simulink model "Pole_Placement_Discrete"  (R2020a)
settings: Solver=VariableStepAuto  StartTime=0.0  StopTime=10.0  RelTol=1e-3
values from neighbouring files (symbols this model uses):
  A_c = [0 1;0 0]    [Discrete_pole_placement.m]
  B_c = [0;K]    [Discrete_pole_placement.m]
  C_c = [1 0]    [Discrete_pole_placement.m]
  Con = 1    [Discrete_pole_placement.m]    (also in Pole_Placement_Integrator.m = 0; Pole_Placement_PID.m = 0)
  D_c = 0    [Discrete_pole_placement.m]
  down = -up    (= -0.10471975512)    [Discrete_pole_placement.m]    (also in Pole_Placement_PID.m = -0.0872664625997)
  K1 = place(A_d,B_d,p_d)    [Discrete_pole_placement.m]    (also in Pole_Placement_Integrator.m = place([A zeros(2,1);-C 0],[B;0],p); Pole_Placement_PID.m = 6.1486)
  L = (A_d^2+sum*A_d+prod*eye(2))*(OBS_d)^(-1)*[0;1]    [Discrete_pole_placement.m]    (also in Pole_Placement_Integrator.m = (A^2+100*A+2500*eye(2))*OBS^(-1)*[0;1])
  steady = D_d+C_d*(eye(2)-(A_d-B_d*K1))^(-1)*B_d    [Discrete_pole_placement.m]
  Ts = 0.02    [Discrete_pole_placement.m]    (also in Pole_Placement_PID.m)
  up = 6*pi/180    (= 0.10471975512)    [Discrete_pole_placement.m]    (also in Pole_Placement_PID.m = 0.0872664625997)
  x0 = 0.1    [Discrete_pole_placement.m]    (also in Pole_Placement_Integrator.m = 0.3; Pole_Placement_PID.m = 0.3)
  y0 = 0.15    [Discrete_pole_placement.m]    (also in Pole_Placement_Integrator.m = 0.3; Pole_Placement_PID.m = 0.3)
undefined symbols (not defined in the file or in its folder): A_d, B_d, C_d
settings Model: Creator=Ashraf  LastModifiedBy=hhiastt
settings DataIOCC: ReturnWorkspaceOutputs=off
settings DebuggingCC: ArithmeticOperatorsInVariantConditions=warning
settings SFSimCC: SimUseLocalCustomCode=off  CustomCodeUndefinedFunction=UseInterfaceOnly
settings RTWCC: RTWUseLocalCustomCode=off
settings CodeAppCC: StateflowObjectComments=on

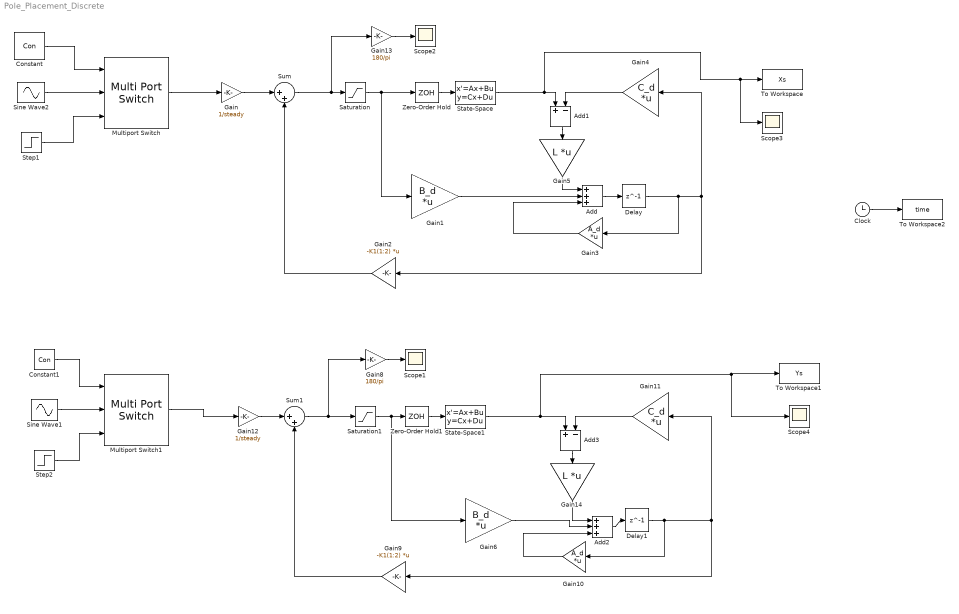
== system Pole_Placement_Discrete ==
  Add : Sum  Inputs=+++
  Add1 : Sum  Inputs=+-
  Add2 : Sum  Inputs=+++
  Add3 : Sum  Inputs=+-
  Clock : Clock
  Constant : Constant  Value=Con
  Constant1 : Constant  Value=Con
  Delay : Delay  DelayLength=1  SampleTime=Ts
  Delay1 : Delay  DelayLength=1  SampleTime=Ts
  Gain : Gain  Gain=1/steady
  Gain1 : Gain  Gain=B_d  Multiplication=Matrix(K*u)
  Gain10 : Gain  Gain=A_d  Multiplication=Matrix(K*u)
  Gain11 : Gain  Gain=C_d  Multiplication=Matrix(K*u)
  Gain12 : Gain  Gain=1/steady
  Gain13 : Gain  Gain=180/pi
  Gain14 : Gain  Gain=L  Multiplication=Matrix(K*u)
  Gain2 : Gain  Gain=-K1(1:2)  Multiplication=Matrix(K*u)
  Gain3 : Gain  Gain=A_d  Multiplication=Matrix(K*u)
  Gain4 : Gain  Gain=C_d  Multiplication=Matrix(K*u)
  Gain5 : Gain  Gain=L  Multiplication=Matrix(K*u)
  Gain6 : Gain  Gain=B_d  Multiplication=Matrix(K*u)
  Gain8 : Gain  Gain=180/pi
  Gain9 : Gain  Gain=-K1(1:2)  Multiplication=Matrix(K*u)
  Multiport Switch : MultiPortSwitch  DataPortOrder=Zero-based contiguous  Inputs=2  zeroidx=on
  Multiport Switch1 : MultiPortSwitch  DataPortOrder=Zero-based contiguous  Inputs=2  zeroidx=on
  Saturation : Saturate  UpperLimit=up  LowerLimit=down
  Saturation1 : Saturate  UpperLimit=up  LowerLimit=down
  Scope{1..4} (4 alike) : Scope
  Sine Wave1 : Sin  Amplitude=0.3  SampleTime=0
  Sine Wave2 : Sin  Amplitude=0.3  Phase=pi/2  SampleTime=Ts
  State-Space : StateSpace  A=A_c  B=B_c  C=C_c  D=D_c  InitialCondition=0
  State-Space1 : StateSpace  A=A_c  B=B_c  C=C_c  D=D_c  InitialCondition=0
  Step1 : Step  Time=0  After=x0  SampleTime=Ts
  Step2 : Step  Time=0  After=y0  SampleTime=0
  Sum : Sum  Inputs=|++
  Sum1 : Sum  Inputs=|++
  To Workspace : ToWorkspace  VariableName=Xs  SampleTime=-1
  To Workspace1 : ToWorkspace  VariableName=Ys  SampleTime=-1
  To Workspace2 : ToWorkspace  VariableName=time  SampleTime=-1
  Zero-Order Hold : ZeroOrderHold  SampleTime=-1
  Zero-Order Hold1 : ZeroOrderHold  SampleTime=-1
  wires:
  Gain2/1 -> Sum/2
  Delay/1 -> Gain4/1, Gain2/1, Gain3/1
  Add/1 -> Delay/1
  Gain4/1 -> Add1/2
  Add1/1 -> Gain5/1
  Gain1/1 -> Add/2
  Gain3/1 -> Add/3
  Clock/1 -> To Workspace2/1
  Sine Wave2/1 -> Multiport Switch/2
  Step1/1 -> Multiport Switch/3
  Constant/1 -> Multiport Switch/1
  Gain13/1 -> Scope2/1
  Multiport Switch/1 -> Gain/1
  State-Space/1 -> Scope3/1, To Workspace/1, Add1/1
  Sum/1 -> Saturation/1, Gain13/1
  Gain9/1 -> Sum1/2
  Delay1/1 -> Gain11/1, Gain9/1, Gain10/1
  Add2/1 -> Delay1/1
  Gain11/1 -> Add3/2
  Add3/1 -> Gain14/1
  Gain14/1 -> Add2/1
  Gain6/1 -> Add2/2
  Gain10/1 -> Add2/3
  Sine Wave1/1 -> Multiport Switch1/2
  Step2/1 -> Multiport Switch1/3
  Constant1/1 -> Multiport Switch1/1
  Gain8/1 -> Scope1/1
  Sum1/1 -> Saturation1/1, Gain8/1
  Gain/1 -> Sum/1
  Zero-Order Hold/1 -> State-Space/1
  Multiport Switch1/1 -> Gain12/1
  Gain12/1 -> Sum1/1
  Zero-Order Hold1/1 -> State-Space1/1
  State-Space1/1 -> Scope4/1, To Workspace1/1, Add3/1
  Saturation/1 -> Zero-Order Hold/1, Gain1/1
  Saturation1/1 -> Zero-Order Hold1/1, Gain6/1
  Gain5/1 -> Add/1
